simulink model "dianya"  (R2023a)
settings: Solver=VariableStepAuto  StartTime=0.0  StopTime=10.0  RelTol=1e-3
settings Model: Creator=Administrator  LastModifiedBy=Administrator

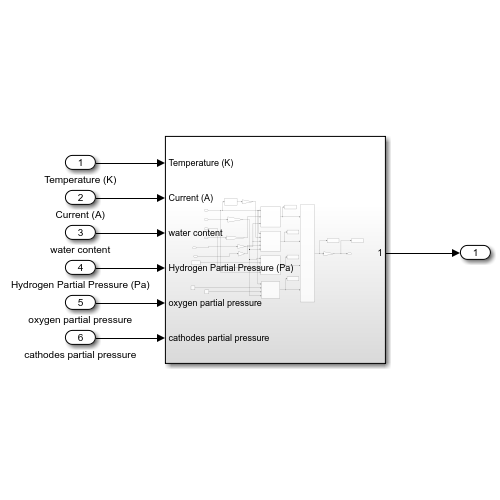
[thumbnail: Simulink's stored preview of the top-level diagram]
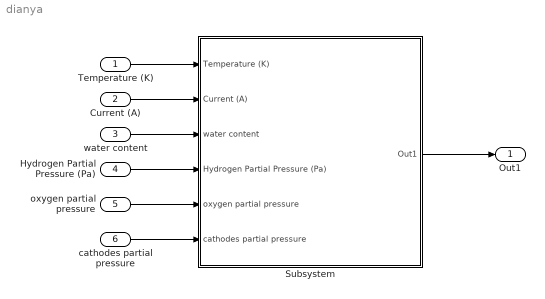
== system dianya ==
  Temperature (K) : Inport
  Current (A) : Inport  Port=2
  water content : Inport  Port=3
  Hydrogen Partial Pressure (Pa) : Inport  Port=4
  oxygen partial pressure : Inport  Port=5
  cathodes partial pressure : Inport  Port=6
  Subsystem : Subsystem
  Out1 : Outport
  wires:
  Temperature (K)/1 -> Subsystem/1(Temperature (K))
  Current (A)/1 -> Subsystem/2(Current (A))
  water content/1 -> Subsystem/3(water content)
  Hydrogen Partial Pressure (Pa)/1 -> Subsystem/4(Hydrogen Partial Pressure (Pa))
  oxygen partial pressure/1 -> Subsystem/5(oxygen partial pressure)
  cathodes partial pressure/1 -> Subsystem/6(cathodes partial pressure)
  Subsystem/1(Out1) -> Out1/1

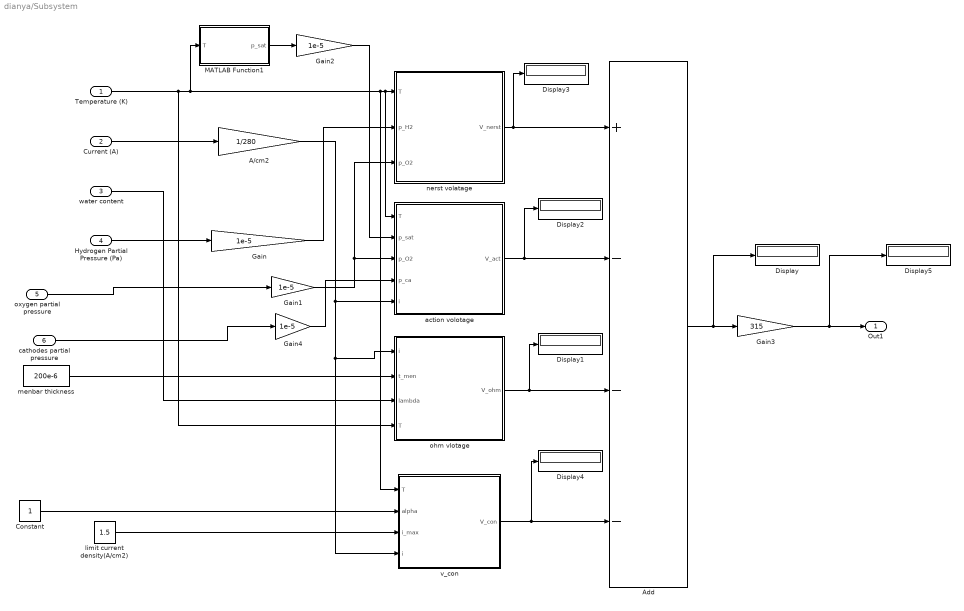
== system dianya/Subsystem ==
  Temperature (K) : Inport
  Current (A) : Inport  Port=2
  water content : Inport  Port=3
  Hydrogen Partial Pressure (Pa) : Inport  Port=4
  oxygen partial pressure : Inport  Port=5
  cathodes partial pressure : Inport  Port=6
  A/cm2 : Gain  Gain=1/280
  Add : Sum  Inputs=+---
  Constant : Constant
  Display{,1..5} (6 alike) : Display
  Gain{,1..2,4} (4 alike) : Gain  Gain=1e-5
  Gain3 : Gain  Gain=315
  MATLAB Function1 : MATLAB Function  TreatAsAtomicUnit=on
  action volotage : MATLAB Function  TreatAsAtomicUnit=on
  limit current density(A/cm2) : Constant  Value=1.5
  menbar thickness : Constant  Value=200e-6
  nerst volatage : MATLAB Function  TreatAsAtomicUnit=on
  ohm vlotage : MATLAB Function  TreatAsAtomicUnit=on
  v_con : MATLAB Function  TreatAsAtomicUnit=on
  Out1 : Outport
  wires:
  action volotage/1(V_act) -> Display2/1, Add/2
  nerst volatage/1(V_nerst) -> Add/1, Display3/1
  A/cm2/1 -> action volotage/5(i), ohm vlotage/1(i), v_con/4(i)
  limit current density(A/cm2)/1 -> v_con/3(i_max)
  oxygen partial pressure/1 -> Gain1/1
  Gain3/1 -> Out1/1, Display5/1
  Temperature (K)/1 -> ohm vlotage/4(T), MATLAB Function1/1(T), action volotage/1(T), nerst volatage/1(T), v_con/1(T)
  Add/1 -> Display/1, Gain3/1
  Constant/1 -> v_con/2(alpha)
  Hydrogen Partial Pressure (Pa)/1 -> Gain/1
  Gain4/1 -> action volotage/4(p_ca)
  menbar thickness/1 -> ohm vlotage/2(t_men)
  Gain1/1 -> action volotage/3(p_O2), nerst volatage/3(p_O2)
  ohm vlotage/1(V_ohm) -> Display1/1, Add/3
  MATLAB Function1/1(p_sat) -> Gain2/1
  water content/1 -> ohm vlotage/3(lambda)
  Gain2/1 -> action volotage/2(p_sat)
  Current (A)/1 -> A/cm2/1
  Gain/1 -> nerst volatage/2(p_H2)
  cathodes partial pressure/1 -> Gain4/1
  v_con/1(V_con) -> Display4/1, Add/4

== matlab function dianya/Subsystem/MATLAB Function1 ==
  data: T input; p_sat output
function p_sat = fcn(T)
p_sat = exp(23.196-3816.44/(T-46.13));

== matlab function dianya/Subsystem/action volotage ==
  data: T input; V_act output; p_sat input; p_O2 input; p_ca input; i input
function V_act = fcn(T,p_sat,p_O2,p_ca,i)
c = 5;
V0 = 0.279-8.5e-4*(T-298.15)+4.308e-4*T*(log((p_ca-p_sat)/1.0135)+0.5*log(0.1173*(p_ca-p_sat)/1.01325));
Va = (-1.618e-5*T+1.618e-2)*(p_O2/0.1173+p_sat)^2+(1.8e-4*T-0.166)*(p_O2/0.1173+p_sat)+(-5.8e-4*T+0.5736);
V_act = V0+Va*(1-exp(-c*i));

== matlab function dianya/Subsystem/nerst volatage ==
  data: T input; V_nerst output; p_H2 input; p_O2 input
function V_nerst = fcn(T,p_H2,p_O2)
V_nerst = 1.229-8.5e-4*(T-298.15)+4.3085e-5*T*(log(p_H2)+0.5*log(p_O2));

== matlab function dianya/Subsystem/ohm vlotage ==
  data: i input; t_men input; V_ohm output; lambda input; T input
function V_ohm = fcn(i,t_men,lambda,T)
sigma=(0.514*lambda-0.033)*exp(1268*(1/303-1/T));%s/m
R_ohm=1e4*t_men/sigma;%ohm*m2
V_ohm = i*R_ohm;

== matlab function dianya/Subsystem/v_con ==
  data: T input; V_con output; alpha input; i_max input; i input
function V_con = fcn(T,alpha,i_max,i)
B = 8.314*T/2/96485*(1+1/alpha);
V_con = B*log(i_max/(i_max-i));
